simulink model "basic_charging_arm"  (R2022b)
settings: Solver=VariableStepAuto  StartTime=0.0  StopTime=100  RelTol=1e-3
values from neighbouring files (symbols this model uses):
  X = zeros(3,1)    [fk.m]
undefined symbols (not defined in the file or in its folder): Y, Z
libraries: fl_lib x64, fl_ps_legacy_lib x32, nesl_utility x25, sm_lib x24, simulink_extras x8, ee_lib x8, simulink x4, slpidlib x4, robotcorelib x1, robotmaniplib x1
(part 1 of 3)
settings Model: Creator=Mohit  LastModifiedBy=Mohit

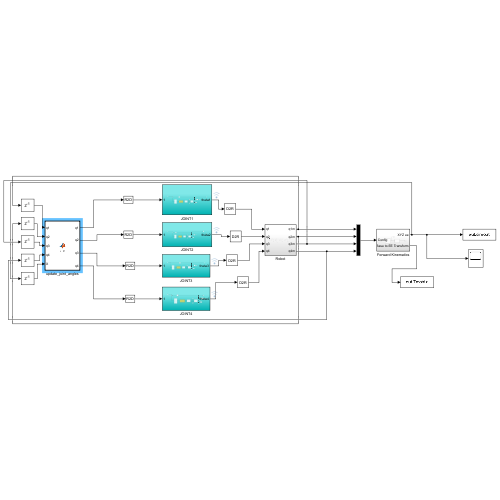
[thumbnail: Simulink's stored preview of the top-level diagram]
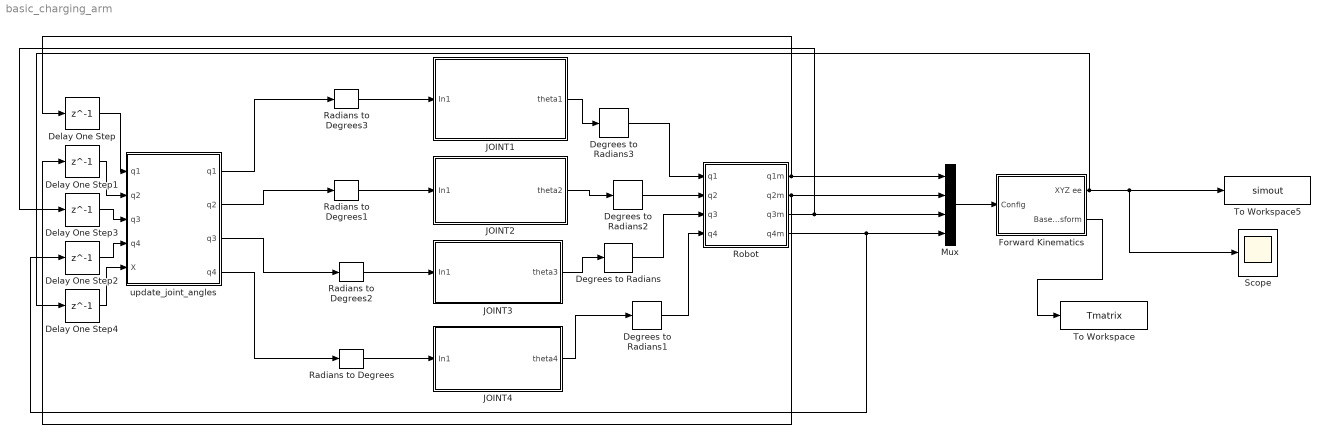
== system basic_charging_arm ==
  Degrees to Radians{,1..3} (4 alike) : simulink_extras/Transformations/Degrees to Radians
  Delay One Step{,1..4} (5 alike) : Delay  DelayLength=1
  Forward Kinematics : Subsystem
  JOINT1 : Subsystem
  JOINT2 : Subsystem
  JOINT3 : Subsystem
  JOINT4 : Subsystem
  Mux : Mux
  Radians to Degrees{,1..3} (4 alike) : simulink_extras/Transformations/Radians to Degrees
  Robot : Subsystem
  Scope : Scope
  To Workspace : ToWorkspace  VariableName=Tmatrix  SaveFormat=Timeseries  SampleTime=-1
  To Workspace5 : ToWorkspace  VariableName=simout  SaveFormat=Timeseries  SampleTime=-1
  update_joint_angles : MATLAB Function  TreatAsAtomicUnit=on
  wires:
  Mux/1 -> Forward Kinematics/1(Config)
  Forward Kinematics/2(Base to EE Transform) -> To Workspace/1
  Robot/1(q1m) -> Delay One Step/1, Mux/1
  Robot/2(q2m) -> Delay One Step1/1, Mux/2
  Robot/3(q3m) -> Delay One Step3/1, Mux/3
  Robot/4(q4m) -> Delay One Step2/1, Mux/4
  Radians to Degrees/1 -> JOINT4/1(In1)
  Radians to Degrees1/1 -> JOINT2/1(In1)
  Radians to Degrees3/1 -> JOINT1/1(In1)
  JOINT1/1(theta1) -> Degrees to Radians3/1
  Forward Kinematics/1(XYZ ee) -> Delay One Step4/1, To Workspace5/1, Scope/1
  JOINT3/1(theta3) -> Degrees to Radians/1
  JOINT4/1(theta4) -> Degrees to Radians1/1
  Radians to Degrees2/1 -> JOINT3/1(In1)
  JOINT2/1(theta2) -> Degrees to Radians2/1
  Degrees to Radians1/1 -> Robot/4(q4)
  Degrees to Radians3/1 -> Robot/1(q1)
  Degrees to Radians2/1 -> Robot/2(q2)
  Degrees to Radians/1 -> Robot/3(q3)
  update_joint_angles/1(q1) -> Radians to Degrees3/1
  update_joint_angles/2(q2) -> Radians to Degrees1/1
  update_joint_angles/3(q3) -> Radians to Degrees2/1
  update_joint_angles/4(q4) -> Radians to Degrees/1
  Delay One Step/1 -> update_joint_angles/1("q1 ")
  Delay One Step2/1 -> update_joint_angles/4("q4 ")
  Delay One Step3/1 -> update_joint_angles/3("q3 ")
  Delay One Step1/1 -> update_joint_angles/2("q2 ")
  Delay One Step4/1 -> update_joint_angles/5(X)

== system basic_charging_arm/Forward Kinematics ==
  Config : Inport
  Coordinate Transformation Conversion : robotcorelib/Coordinate Transformation Conversion  InputRepresentation=Homogeneous Transformation  InputEulerSequence=ZYX  ShowTrVecInputPort=on  OutputRepresentation=Translation Vector  OutputEulerSequence=ZYX  ShowTrVecOutputPort=on  SimulateUsing=Interpreted execution
  Get Transform : robotmaniplib/Get Transform  RigidBodyTree=Basic_arm_rbt  SourceBody=Body5  TargetBody=Base  SimulateUsing=Interpreted execution
  XYZ ee : Outport
  Base to EE Transform : Outport  Port=2
  wires:
  Config/1 -> Get Transform/1
  Coordinate Transformation Conversion/1 -> XYZ ee/1  "XYZ ee"
  Get Transform/1 -> Base to EE Transform/1, Coordinate Transformation Conversion/1

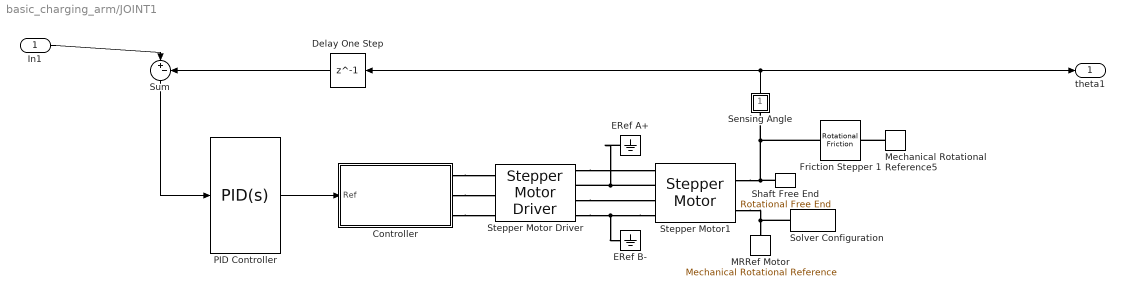
== system basic_charging_arm/JOINT1 ==
  In1 : Inport
  Controller : Subsystem  Variant=on  VariantControlMode=label  LabelModeActiveChoice=Speed
      settings: AttributesFormatString=%<BlockChoice>
  Delay One Step : Delay  DelayLength=1
  ERef A+ : fl_lib/Electrical/Electrical Elements/Electrical Reference
  ERef B- : fl_lib/Electrical/Electrical Elements/Electrical Reference
  Friction Stepper 1 : fl_lib/Mechanical/Rotational Elements/Rotational Friction  brkwy_trq=3.0e-2 N*m  brkwy_vel=0.03347 rad/s  Col_trq=3.0e-2 N*m  visc_coef=0 N*m/(rad/s)  w_specify=off  w_priority=High  w=0 rad/s  w_nominal_specify=off  w_nominal_unit=rad/s  w_nominal_value=1  t_specify=off  t_priority=High  t=0 N*m  t_nominal_specify=off  t_nominal_unit=N*m  t_nominal_value=1
  MRRef Motor : fl_lib/Mechanical/Rotational Elements/Mechanical Rotational Reference
  Mechanical Rotational Reference5 : fl_lib/Mechanical/Rotational Elements/Mechanical Rotational Reference
  PID Controller : slpidlib/PID Controller  Controller=PID  Form=Parallel  TimeDomain=Continuous-time  UseExternalTs=off  SampleTime=-1  IntegratorMethod=Forward Euler  FilterMethod=Forward Euler  ControllerParametersSource=internal  P=6  I=6  UseKiTs=off  D=0  N=100  UseFilter=on  TunerSelectOption=Transfer Function Based (PID Tuner App)  InitialConditionSource=internal  InitialConditionForIntegrator=0  InitialConditionForFilter=0  DifferentiatorICPrevScaledInput=0  ExternalReset=none  TrackingMode=off  Kt=1  LimitOutput=off  SatLimitsSource=internal  UpperSaturationLimit=inf  LowerSaturationLimit=-inf  LinearizeAsGain=on  AntiWindupMode=none  Kb=1  LimitIntegrator=off  UpperIntegratorSaturationLimit=inf  LowerIntegratorSaturationLimit=-inf  POutMin=[]  POutMax=[]  IOutMin=[]  IOutMax=[]  DOutMin=[]  DOutMax=[]  NOutMin=[]  NOutMax=[]  SumOutMin=[]  SumOutMax=[]  SaturationOutMin=[]  SaturationOutMax=[]  PParamMin=[]  PParamMax=[]  IParamMin=[]  IParamMax=[]  DParamMin=[]  DParamMax=[]  NParamMin=[]  NParamMax=[]  KbParamMin=[]  KbParamMax=[]  KtParamMin=[]  KtParamMax=[]  KbOutMin=[]  KbOutMax=[]  KtOutMin=[]  KtOutMax=[]  IntegratorOutMin=[]  IntegratorOutMax=[]  FilterOutMin=[]  FilterOutMax=[]  SumI1OutMin=[]  SumI1OutMax=[]  SumI2OutMin=[]  SumI2OutMax=[]  SumI3OutMin=[]  SumI3OutMax=[]  SumI4OutMin=[]  SumI4OutMax=[]  SumDOutMin=[]  SumDOutMax=[]  DifferentiatorOutMin=[]  DifferentiatorOutMax=[]  FilterDiffOutCoefMin=[]  FilterDiffOutCoefMax=[]  ReciprocalOutMin=[]  ReciprocalOutMax=[]  SumDenOutMin=[]  SumDenOutMax=[]  SumNumOutMin=[]  SumNumOutMax=[]  DivideOutMin=[]  DivideOutMax=[]  UdiffTsProdOutMin=[]  UdiffTsProdOutMax=[]  NTsProdOutMin=[]  NTsProdOutMax=[]  UintegralTsProdOutMin=[]  UintegralTsProdOutMax=[]  UngainTsProdOutMin=[]  UngainTsProdOutMax=[]  ClampingZeroOutDataTypeStr=Inherit: Inherit via back propagation  ClampingZeroOutMin=[]  ClampingZeroOutMax=[]  FilterDenConstantOutDataTypeStr=Inherit: Inherit via back propagation  FilterDenConstantOutMin=[]  FilterDenConstantOutMax=[]  PCopyOutDataTypeStr=Inherit: Inherit via back propagation  PCopyOutMin=[]  PCopyOutMax=[]  NCopyOutDataTypeStr=Inherit: Inherit via back propagation  NCopyOutMin=[]  NCopyOutMax=[]  IntegratorContinuousStateAttributes=''  IntegratorStateMustResolveToSignalObject=off  IntegratorRTWStateStorageClass=Auto  FilterContinuousStateAttributes=''  FilterStateMustResolveToSignalObject=off  FilterRTWStateStorageClass=Auto  ParallelPVariant=InternalParameters  IdealPVariant=Disabled  IVariant=InternalParameters  DVariant=InternalParameters  IntegratorVariant=Continuous  SatVariant=Disabled  AWVariant=Passthrough  PCopyVariant=Disabled  TRVariant=Disabled  FdbkBlocksVariant=Forward  IdealPFdbkVariant=Disabled  SatFdbkVariant=Disabled  DerivativeFilterVariant=ContFilter  NVariant=InternalParameters  NCopyVariant=Disabled  FilterICVariant=InternalICsFilter  IntegratorICVariant=InternalICs  ExternalResetVariant=Disabled  TRSumVariant=Passthrough  SumFdbkVariant=Disabled  SumVariant=Sum_PID  TsampFilterVariant=InternalTs  TsampNgainVariant=Passthrough  TsampIntegralVariant=Passthrough  ExternalSaturationOutDataTypeStr=Inherit: Same as second input
  Sensing Angle : Subsystem
      mask Display: disp('a')
  Shaft Free End : fl_lib/Mechanical/Rotational Elements/Rotational Free End  w_specify=off  w_priority=None  w=0 rad/s  w_nominal_specify=off  w_nominal_unit=rad/s  w_nominal_value=1
  Solver Configuration : nesl_utility/Solver Configuration  PhysicalDomain=network_engine_domain  SubClassName=solver  LeftPortType=input  RightPortType=generic  Tones=[]  Harmonics=[]  SimulateNoise=off  Profile=off  UseLocalSampling=off  EnableSwitchedLinearOptims=on  FrequencyDomain=off  UseCCode=off  RelTol=0.001  AbsTol=1e-06  MinStep=1e-09  ToWorkspace=off  RevertToSquareIcSolve=off  NumHomotopyIterations=100  PhasorMode=off  PhasorModeNumHarmonics=1  ConsistencySolver=NEWTON_FTOL  IndexReductionMethod=DerivativeReplacement  DoDC=off  ResidualTolerance=1e-9  ConsistencyTolSource=GLOBAL  ConsistencyAbsTol=0.001  ConsistencyRelTol=0.001  ConsistencyTolFactor=0.001  UseLocalSolver=off  LocalSolverChoice=NE_BACKWARD_EULER_ADVANCER  ResolveIndetEquations=on  FunctionEvalNumThread=1  LocalSolverSampleTime=.001  DoFixedCost=off  MaxNonlinIter=3  MaxModeIter=2  ComputeImpulses=off  ImpulseIterations=2  LinearAlgebra=auto  LinearAlgebraNumThread=0  EquationFormulation=NE_TIME_EF  DelaysMemoryBudget=1024  AutomaticFiltering=on  FilteringTimeConstant=0.001  PartitionStorageMethod=AS_NEEDED  PartitionMemoryBudget=1024  PartitionMethod=FAST
  Stepper Motor Driver : ee_lib/Electromechanical/Reluctance & Stepper/Stepper Motor Driver  step_or_av=ee.enum.electromech.simulationMode.stepping  step_rate_per_volt=10 Hz/V  Venable=2.5 V  Vreverse=2.5 V  supply_ports=ee.enum.supply_ports.hidesupply  Vm=5 V  Vsupply=10 V  half_stepping=ee.enum.electromech.steppingModeAveraged.fullStep  stepping_mode=ee.enum.electromech.steppingMode.microStep  numMicroSteps=4  Im=1.2 A
      settings: InternalSimscapePortConfiguration="{\"Bottom\":[],\"Left\":[{\"id\":\"ENA\",\"label\":\"ENA\",\"type\":\"foundation.electrical.electrical\"},{\"id\":\"REF\",\"label\":\"REF\",\"type\":\"foundation.electrical.electrical\"},{\"id\":\"REV\",\"label\":\"REV\",\"type\":\"foundation.electrical.electrical\"}],\"Right\":[{\"id\":\"pA\",\"label\":\"A+\",\"type\":\"foundation.electrical.electrical\"},{\"id\":\"nA\",\"label\":\"A-\",\"type\":\"foundation.electrical.electrical\"},{\"id\":\"pB\",\"label\":\"B+\",\"type\":\"foundation.electrical.electrical\"},{\"id\":\"nB\",\"label\":\"B-\",\"type\":\"foundation.electrical.electrical\"}],\"Top\":[]}"
  Stepper Motor1 : ee_lib/Electromechanical/Reluctance & Stepper/Stepper Motor  step_or_av=1  Ra=0.55 Ohm  La=0.0015 H  Km=0.19 N*m/A  Td=0 N*m  Rm=Inf Ohm  w_vec=[ 0 1000 3e+3 ] rpm  T_vec=[ 2 2 1 ] N*m  assert_if_slipping=0  J_total=1e-4 kg*m^2  max_step_rate=10 Hz  Step=1.8 deg  J=4.5e-05 kg*m^2  B=1e-02 N*m/(rad/s)  speed0=0 rpm  theta0=0 deg  alpha=[.00393, .00393] 1/K  Tmeas=25 degC  Tmeas2=125 degC  T_vec2=[1.7, 1.7, .85] N*m  half_stepping=ee.enum.electromech.steppingModeAveraged.fullStep  thermal_masses=[100, 100] J/K  initial_temperatures=[25, 25] degC  rotor_thermal_mass=50 J/K  rotor_initial_temperature=25 degC  Rm_percent_rotor=90
      settings: InternalSimscapePortConfiguration="{\"Bottom\":[],\"Left\":[{\"id\":\"pA\",\"label\":\"A+\",\"type\":\"foundation.electrical.electrical\"},{\"id\":\"nA\",\"label\":\"A-\",\"type\":\"foundation.electrical.electrical\"},{\"id\":\"pB\",\"label\":\"B+\",\"type\":\"foundation.electrical.electrical\"},{\"id\":\"nB\",\"label\":\"B-\",\"type\":\"foundation.electrical.electrical\"}],\"Right\":[{\"id\":\"R\",\"label\":\"R\",\"type\":\"foundation.mechanical.rotational.rotational\"},{\"id\":\"C\",\"label\":\"C\",\"type\":\"foundation.mechanical.rotational.rotational\"}],\"Top\":[]}"
  Sum : Sum  Inputs=|+-
  theta1 : Outport
  wires:
  In1/1 -> Sum/1
  Sum/1 -> PID Controller/1
  Sensing Angle/1(theta) -> theta1/1, Delay One Step/1
  PID Controller/1 -> Controller/1(Ref)
  Delay One Step/1 -> Sum/2
  connections:
  Controller/RConn2 -- Stepper Motor Driver/LConn2
  Stepper Motor Driver/RConn1 -- Stepper Motor1/LConn1
  Controller/RConn1 -- Stepper Motor Driver/LConn1
  Solver Configuration/RConn1 -- Stepper Motor1/RConn2 -- MRRef Motor/LConn1
  ERef A+/LConn1 -- Stepper Motor1/LConn2 -- Stepper Motor Driver/RConn2
  Stepper Motor Driver/RConn3 -- Stepper Motor1/LConn3
  Mechanical Rotational Reference5/LConn1 -- Friction Stepper 1/RConn1
  Controller/RConn3 -- Stepper Motor Driver/LConn3
  Stepper Motor1/LConn4 -- Stepper Motor Driver/RConn4 -- ERef B-/LConn1
  Sensing Angle/LConn1 -- Friction Stepper 1/LConn1 -- Shaft Free End/LConn1 -- Stepper Motor1/RConn1

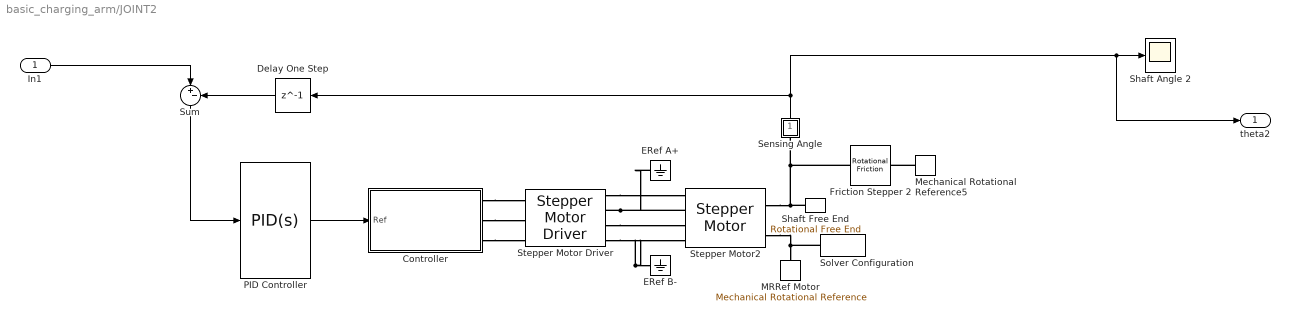
== system basic_charging_arm/JOINT2 ==
  In1 : Inport
  Controller : Subsystem  Variant=on  VariantControlMode=label  LabelModeActiveChoice=Speed
      settings: AttributesFormatString=%<BlockChoice>
  Delay One Step : Delay  DelayLength=1
  ERef A+ : fl_lib/Electrical/Electrical Elements/Electrical Reference
  ERef B- : fl_lib/Electrical/Electrical Elements/Electrical Reference
  Friction Stepper 2 : fl_lib/Mechanical/Rotational Elements/Rotational Friction  brkwy_trq=3.0e-2 N*m  brkwy_vel=0.03347 rad/s  Col_trq=3.0e-2 N*m  visc_coef=0 N*m/(rad/s)  w_specify=off  w_priority=High  w=0 rad/s  w_nominal_specify=off  w_nominal_unit=rad/s  w_nominal_value=1  t_specify=off  t_priority=High  t=0 N*m  t_nominal_specify=off  t_nominal_unit=N*m  t_nominal_value=1
  MRRef Motor : fl_lib/Mechanical/Rotational Elements/Mechanical Rotational Reference
  Mechanical Rotational Reference5 : fl_lib/Mechanical/Rotational Elements/Mechanical Rotational Reference
  PID Controller : slpidlib/PID Controller  Controller=PID  Form=Parallel  TimeDomain=Continuous-time  UseExternalTs=off  SampleTime=-1  IntegratorMethod=Forward Euler  FilterMethod=Forward Euler  ControllerParametersSource=internal  P=6  I=6  UseKiTs=off  D=0  N=100  UseFilter=on  TunerSelectOption=Transfer Function Based (PID Tuner App)  InitialConditionSource=internal  InitialConditionForIntegrator=0  InitialConditionForFilter=0  DifferentiatorICPrevScaledInput=0  ExternalReset=none  TrackingMode=off  Kt=1  LimitOutput=off  SatLimitsSource=internal  UpperSaturationLimit=inf  LowerSaturationLimit=-inf  LinearizeAsGain=on  AntiWindupMode=none  Kb=1  LimitIntegrator=off  UpperIntegratorSaturationLimit=inf  LowerIntegratorSaturationLimit=-inf  POutMin=[]  POutMax=[]  IOutMin=[]  IOutMax=[]  DOutMin=[]  DOutMax=[]  NOutMin=[]  NOutMax=[]  SumOutMin=[]  SumOutMax=[]  SaturationOutMin=[]  SaturationOutMax=[]  PParamMin=[]  PParamMax=[]  IParamMin=[]  IParamMax=[]  DParamMin=[]  DParamMax=[]  NParamMin=[]  NParamMax=[]  KbParamMin=[]  KbParamMax=[]  KtParamMin=[]  KtParamMax=[]  KbOutMin=[]  KbOutMax=[]  KtOutMin=[]  KtOutMax=[]  IntegratorOutMin=[]  IntegratorOutMax=[]  FilterOutMin=[]  FilterOutMax=[]  SumI1OutMin=[]  SumI1OutMax=[]  SumI2OutMin=[]  SumI2OutMax=[]  SumI3OutMin=[]  SumI3OutMax=[]  SumI4OutMin=[]  SumI4OutMax=[]  SumDOutMin=[]  SumDOutMax=[]  DifferentiatorOutMin=[]  DifferentiatorOutMax=[]  FilterDiffOutCoefMin=[]  FilterDiffOutCoefMax=[]  ReciprocalOutMin=[]  ReciprocalOutMax=[]  SumDenOutMin=[]  SumDenOutMax=[]  SumNumOutMin=[]  SumNumOutMax=[]  DivideOutMin=[]  DivideOutMax=[]  UdiffTsProdOutMin=[]  UdiffTsProdOutMax=[]  NTsProdOutMin=[]  NTsProdOutMax=[]  UintegralTsProdOutMin=[]  UintegralTsProdOutMax=[]  UngainTsProdOutMin=[]  UngainTsProdOutMax=[]  ClampingZeroOutDataTypeStr=Inherit: Inherit via back propagation  ClampingZeroOutMin=[]  ClampingZeroOutMax=[]  FilterDenConstantOutDataTypeStr=Inherit: Inherit via back propagation  FilterDenConstantOutMin=[]  FilterDenConstantOutMax=[]  PCopyOutDataTypeStr=Inherit: Inherit via back propagation  PCopyOutMin=[]  PCopyOutMax=[]  NCopyOutDataTypeStr=Inherit: Inherit via back propagation  NCopyOutMin=[]  NCopyOutMax=[]  IntegratorContinuousStateAttributes=''  IntegratorStateMustResolveToSignalObject=off  IntegratorRTWStateStorageClass=Auto  FilterContinuousStateAttributes=''  FilterStateMustResolveToSignalObject=off  FilterRTWStateStorageClass=Auto  ParallelPVariant=InternalParameters  IdealPVariant=Disabled  IVariant=InternalParameters  DVariant=InternalParameters  IntegratorVariant=Continuous  SatVariant=Disabled  AWVariant=Passthrough  PCopyVariant=Disabled  TRVariant=Disabled  FdbkBlocksVariant=Forward  IdealPFdbkVariant=Disabled  SatFdbkVariant=Disabled  DerivativeFilterVariant=ContFilter  NVariant=InternalParameters  NCopyVariant=Disabled  FilterICVariant=InternalICsFilter  IntegratorICVariant=InternalICs  ExternalResetVariant=Disabled  TRSumVariant=Passthrough  SumFdbkVariant=Disabled  SumVariant=Sum_PID  TsampFilterVariant=InternalTs  TsampNgainVariant=Passthrough  TsampIntegralVariant=Passthrough  ExternalSaturationOutDataTypeStr=Inherit: Same as second input
  Sensing Angle : Subsystem
      mask Display: disp('a')
  Shaft Angle 2 : Scope
  Shaft Free End : fl_lib/Mechanical/Rotational Elements/Rotational Free End  w_specify=off  w_priority=None  w=0 rad/s  w_nominal_specify=off  w_nominal_unit=rad/s  w_nominal_value=1
  Solver Configuration : nesl_utility/Solver Configuration  PhysicalDomain=network_engine_domain  SubClassName=solver  LeftPortType=input  RightPortType=generic  Tones=[]  Harmonics=[]  SimulateNoise=off  Profile=off  UseLocalSampling=off  EnableSwitchedLinearOptims=on  FrequencyDomain=off  UseCCode=off  RelTol=0.001  AbsTol=1e-06  MinStep=1e-09  ToWorkspace=off  RevertToSquareIcSolve=off  NumHomotopyIterations=100  PhasorMode=off  PhasorModeNumHarmonics=1  ConsistencySolver=NEWTON_FTOL  IndexReductionMethod=DerivativeReplacement  DoDC=off  ResidualTolerance=1e-9  ConsistencyTolSource=GLOBAL  ConsistencyAbsTol=0.001  ConsistencyRelTol=0.001  ConsistencyTolFactor=0.001  UseLocalSolver=off  LocalSolverChoice=NE_BACKWARD_EULER_ADVANCER  ResolveIndetEquations=on  FunctionEvalNumThread=1  LocalSolverSampleTime=.001  DoFixedCost=off  MaxNonlinIter=3  MaxModeIter=2  ComputeImpulses=off  ImpulseIterations=2  LinearAlgebra=auto  LinearAlgebraNumThread=0  EquationFormulation=NE_TIME_EF  DelaysMemoryBudget=1024  AutomaticFiltering=on  FilteringTimeConstant=0.001  PartitionStorageMethod=AS_NEEDED  PartitionMemoryBudget=1024  PartitionMethod=FAST
  Stepper Motor Driver : ee_lib/Electromechanical/Reluctance & Stepper/Stepper Motor Driver  step_or_av=ee.enum.electromech.simulationMode.stepping  step_rate_per_volt=10 Hz/V  Venable=2.5 V  Vreverse=2.5 V  supply_ports=ee.enum.supply_ports.hidesupply  Vm=5 V  Vsupply=10 V  half_stepping=ee.enum.electromech.steppingModeAveraged.fullStep  stepping_mode=ee.enum.electromech.steppingMode.microStep  numMicroSteps=4  Im=1.2 A
      settings: InternalSimscapePortConfiguration="{\"Bottom\":[],\"Left\":[{\"id\":\"ENA\",\"label\":\"ENA\",\"type\":\"foundation.electrical.electrical\"},{\"id\":\"REF\",\"label\":\"REF\",\"type\":\"foundation.electrical.electrical\"},{\"id\":\"REV\",\"label\":\"REV\",\"type\":\"foundation.electrical.electrical\"}],\"Right\":[{\"id\":\"pA\",\"label\":\"A+\",\"type\":\"foundation.electrical.electrical\"},{\"id\":\"nA\",\"label\":\"A-\",\"type\":\"foundation.electrical.electrical\"},{\"id\":\"pB\",\"label\":\"B+\",\"type\":\"foundation.electrical.electrical\"},{\"id\":\"nB\",\"label\":\"B-\",\"type\":\"foundation.electrical.electrical\"}],\"Top\":[]}"
  Stepper Motor2 : ee_lib/Electromechanical/Reluctance & Stepper/Stepper Motor  step_or_av=1  Ra=0.55 Ohm  La=0.0015 H  Km=0.19 N*m/A  Td=0 N*m  Rm=Inf Ohm  w_vec=[ 0 1000 3e+3 ] rpm  T_vec=[ 2 2 1 ] N*m  assert_if_slipping=0  J_total=1e-4 kg*m^2  max_step_rate=10 Hz  Step=1.8 deg  J=4.5e-05 kg*m^2  B=1e-02 N*m/(rad/s)  speed0=0 rpm  theta0=0 deg  alpha=[.00393, .00393] 1/K  Tmeas=25 degC  Tmeas2=125 degC  T_vec2=[1.7, 1.7, .85] N*m  half_stepping=ee.enum.electromech.steppingModeAveraged.fullStep  thermal_masses=[100, 100] J/K  initial_temperatures=[25, 25] degC  rotor_thermal_mass=50 J/K  rotor_initial_temperature=25 degC  Rm_percent_rotor=90
      settings: InternalSimscapePortConfiguration="{\"Bottom\":[],\"Left\":[{\"id\":\"pA\",\"label\":\"A+\",\"type\":\"foundation.electrical.electrical\"},{\"id\":\"nA\",\"label\":\"A-\",\"type\":\"foundation.electrical.electrical\"},{\"id\":\"pB\",\"label\":\"B+\",\"type\":\"foundation.electrical.electrical\"},{\"id\":\"nB\",\"label\":\"B-\",\"type\":\"foundation.electrical.electrical\"}],\"Right\":[{\"id\":\"R\",\"label\":\"R\",\"type\":\"foundation.mechanical.rotational.rotational\"},{\"id\":\"C\",\"label\":\"C\",\"type\":\"foundation.mechanical.rotational.rotational\"}],\"Top\":[]}"
  Sum : Sum  Inputs=|+-
  theta2 : Outport
  wires:
  PID Controller/1 -> Controller/1(Ref)
  Sensing Angle/1(theta) -> Delay One Step/1, theta2/1, Shaft Angle 2/1
  Sum/1 -> PID Controller/1
  In1/1 -> Sum/1
  Delay One Step/1 -> Sum/2
  connections:
  Stepper Motor2/RConn1 -- Shaft Free End/LConn1 -- Friction Stepper 2/LConn1 -- Sensing Angle/LConn1
  ERef B-/LConn1 -- Stepper Motor Driver/RConn4 -- Stepper Motor2/LConn4
  Controller/RConn3 -- Stepper Motor Driver/LConn3
  Mechanical Rotational Reference5/LConn1 -- Friction Stepper 2/RConn1
  Stepper Motor Driver/RConn3 -- Stepper Motor2/LConn3
  Stepper Motor Driver/RConn2 -- Stepper Motor2/LConn2 -- ERef A+/LConn1
  MRRef Motor/LConn1 -- Stepper Motor2/RConn2 -- Solver Configuration/RConn1
  Controller/RConn1 -- Stepper Motor Driver/LConn1
  Stepper Motor Driver/RConn1 -- Stepper Motor2/LConn1
  Controller/RConn2 -- Stepper Motor Driver/LConn2

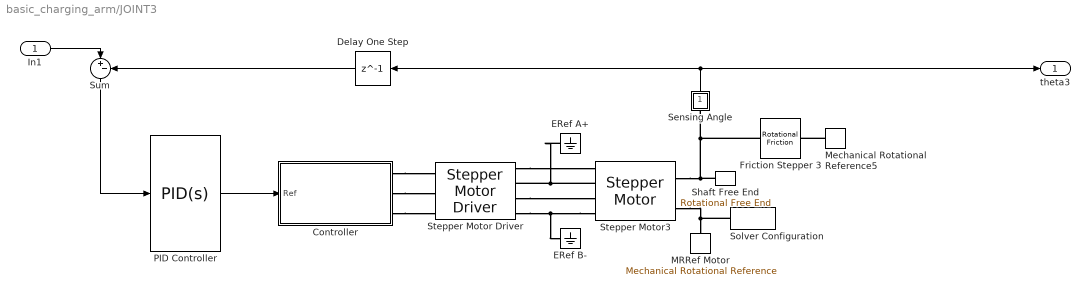
== system basic_charging_arm/JOINT3 ==
  In1 : Inport
  Controller : Subsystem  Variant=on  VariantControlMode=label  LabelModeActiveChoice=Speed
      settings: AttributesFormatString=%<BlockChoice>
  Delay One Step : Delay  DelayLength=1
  ERef A+ : fl_lib/Electrical/Electrical Elements/Electrical Reference
  ERef B- : fl_lib/Electrical/Electrical Elements/Electrical Reference
  Friction Stepper 3 : fl_lib/Mechanical/Rotational Elements/Rotational Friction  brkwy_trq=3.0e-2 N*m  brkwy_vel=0.03347 rad/s  Col_trq=3.0e-2 N*m  visc_coef=0 N*m/(rad/s)  w_specify=off  w_priority=High  w=0 rad/s  w_nominal_specify=off  w_nominal_unit=rad/s  w_nominal_value=1  t_specify=off  t_priority=High  t=0 N*m  t_nominal_specify=off  t_nominal_unit=N*m  t_nominal_value=1
  MRRef Motor : fl_lib/Mechanical/Rotational Elements/Mechanical Rotational Reference
  Mechanical Rotational Reference5 : fl_lib/Mechanical/Rotational Elements/Mechanical Rotational Reference
  PID Controller : slpidlib/PID Controller  Controller=PID  Form=Parallel  TimeDomain=Continuous-time  UseExternalTs=off  SampleTime=-1  IntegratorMethod=Forward Euler  FilterMethod=Forward Euler  ControllerParametersSource=internal  P=6  I=6  UseKiTs=off  D=0  N=100  UseFilter=on  TunerSelectOption=Transfer Function Based (PID Tuner App)  InitialConditionSource=internal  InitialConditionForIntegrator=0  InitialConditionForFilter=0  DifferentiatorICPrevScaledInput=0  ExternalReset=none  TrackingMode=off  Kt=1  LimitOutput=off  SatLimitsSource=internal  UpperSaturationLimit=inf  LowerSaturationLimit=-inf  LinearizeAsGain=on  AntiWindupMode=none  Kb=1  LimitIntegrator=off  UpperIntegratorSaturationLimit=inf  LowerIntegratorSaturationLimit=-inf  POutMin=[]  POutMax=[]  IOutMin=[]  IOutMax=[]  DOutMin=[]  DOutMax=[]  NOutMin=[]  NOutMax=[]  SumOutMin=[]  SumOutMax=[]  SaturationOutMin=[]  SaturationOutMax=[]  PParamMin=[]  PParamMax=[]  IParamMin=[]  IParamMax=[]  DParamMin=[]  DParamMax=[]  NParamMin=[]  NParamMax=[]  KbParamMin=[]  KbParamMax=[]  KtParamMin=[]  KtParamMax=[]  KbOutMin=[]  KbOutMax=[]  KtOutMin=[]  KtOutMax=[]  IntegratorOutMin=[]  IntegratorOutMax=[]  FilterOutMin=[]  FilterOutMax=[]  SumI1OutMin=[]  SumI1OutMax=[]  SumI2OutMin=[]  SumI2OutMax=[]  SumI3OutMin=[]  SumI3OutMax=[]  SumI4OutMin=[]  SumI4OutMax=[]  SumDOutMin=[]  SumDOutMax=[]  DifferentiatorOutMin=[]  DifferentiatorOutMax=[]  FilterDiffOutCoefMin=[]  FilterDiffOutCoefMax=[]  ReciprocalOutMin=[]  ReciprocalOutMax=[]  SumDenOutMin=[]  SumDenOutMax=[]  SumNumOutMin=[]  SumNumOutMax=[]  DivideOutMin=[]  DivideOutMax=[]  UdiffTsProdOutMin=[]  UdiffTsProdOutMax=[]  NTsProdOutMin=[]  NTsProdOutMax=[]  UintegralTsProdOutMin=[]  UintegralTsProdOutMax=[]  UngainTsProdOutMin=[]  UngainTsProdOutMax=[]  ClampingZeroOutDataTypeStr=Inherit: Inherit via back propagation  ClampingZeroOutMin=[]  ClampingZeroOutMax=[]  FilterDenConstantOutDataTypeStr=Inherit: Inherit via back propagation  FilterDenConstantOutMin=[]  FilterDenConstantOutMax=[]  PCopyOutDataTypeStr=Inherit: Inherit via back propagation  PCopyOutMin=[]  PCopyOutMax=[]  NCopyOutDataTypeStr=Inherit: Inherit via back propagation  NCopyOutMin=[]  NCopyOutMax=[]  IntegratorContinuousStateAttributes=''  IntegratorStateMustResolveToSignalObject=off  IntegratorRTWStateStorageClass=Auto  FilterContinuousStateAttributes=''  FilterStateMustResolveToSignalObject=off  FilterRTWStateStorageClass=Auto  ParallelPVariant=InternalParameters  IdealPVariant=Disabled  IVariant=InternalParameters  DVariant=InternalParameters  IntegratorVariant=Continuous  SatVariant=Disabled  AWVariant=Passthrough  PCopyVariant=Disabled  TRVariant=Disabled  FdbkBlocksVariant=Forward  IdealPFdbkVariant=Disabled  SatFdbkVariant=Disabled  DerivativeFilterVariant=ContFilter  NVariant=InternalParameters  NCopyVariant=Disabled  FilterICVariant=InternalICsFilter  IntegratorICVariant=InternalICs  ExternalResetVariant=Disabled  TRSumVariant=Passthrough  SumFdbkVariant=Disabled  SumVariant=Sum_PID  TsampFilterVariant=InternalTs  TsampNgainVariant=Passthrough  TsampIntegralVariant=Passthrough  ExternalSaturationOutDataTypeStr=Inherit: Same as second input
  Sensing Angle : Subsystem
      mask Display: disp('a')
  Shaft Free End : fl_lib/Mechanical/Rotational Elements/Rotational Free End  w_specify=off  w_priority=None  w=0 rad/s  w_nominal_specify=off  w_nominal_unit=rad/s  w_nominal_value=1
  Solver Configuration : nesl_utility/Solver Configuration  PhysicalDomain=network_engine_domain  SubClassName=solver  LeftPortType=input  RightPortType=generic  Tones=[]  Harmonics=[]  SimulateNoise=off  Profile=off  UseLocalSampling=off  EnableSwitchedLinearOptims=on  FrequencyDomain=off  UseCCode=off  RelTol=0.001  AbsTol=1e-06  MinStep=1e-09  ToWorkspace=off  RevertToSquareIcSolve=off  NumHomotopyIterations=100  PhasorMode=off  PhasorModeNumHarmonics=1  ConsistencySolver=NEWTON_FTOL  IndexReductionMethod=DerivativeReplacement  DoDC=off  ResidualTolerance=1e-9  ConsistencyTolSource=GLOBAL  ConsistencyAbsTol=0.001  ConsistencyRelTol=0.001  ConsistencyTolFactor=0.001  UseLocalSolver=off  LocalSolverChoice=NE_BACKWARD_EULER_ADVANCER  ResolveIndetEquations=on  FunctionEvalNumThread=1  LocalSolverSampleTime=.001  DoFixedCost=off  MaxNonlinIter=3  MaxModeIter=2  ComputeImpulses=off  ImpulseIterations=2  LinearAlgebra=auto  LinearAlgebraNumThread=0  EquationFormulation=NE_TIME_EF  DelaysMemoryBudget=1024  AutomaticFiltering=on  FilteringTimeConstant=0.001  PartitionStorageMethod=AS_NEEDED  PartitionMemoryBudget=1024  PartitionMethod=FAST
  Stepper Motor Driver : ee_lib/Electromechanical/Reluctance & Stepper/Stepper Motor Driver  step_or_av=ee.enum.electromech.simulationMode.stepping  step_rate_per_volt=10 Hz/V  Venable=2.5 V  Vreverse=2.5 V  supply_ports=ee.enum.supply_ports.hidesupply  Vm=5 V  Vsupply=10 V  half_stepping=ee.enum.electromech.steppingModeAveraged.fullStep  stepping_mode=ee.enum.electromech.steppingMode.microStep  numMicroSteps=4  Im=1.2 A
      settings: InternalSimscapePortConfiguration="{\"Bottom\":[],\"Left\":[{\"id\":\"ENA\",\"label\":\"ENA\",\"type\":\"foundation.electrical.electrical\"},{\"id\":\"REF\",\"label\":\"REF\",\"type\":\"foundation.electrical.electrical\"},{\"id\":\"REV\",\"label\":\"REV\",\"type\":\"foundation.electrical.electrical\"}],\"Right\":[{\"id\":\"pA\",\"label\":\"A+\",\"type\":\"foundation.electrical.electrical\"},{\"id\":\"nA\",\"label\":\"A-\",\"type\":\"foundation.electrical.electrical\"},{\"id\":\"pB\",\"label\":\"B+\",\"type\":\"foundation.electrical.electrical\"},{\"id\":\"nB\",\"label\":\"B-\",\"type\":\"foundation.electrical.electrical\"}],\"Top\":[]}"
  Stepper Motor3 : ee_lib/Electromechanical/Reluctance & Stepper/Stepper Motor  step_or_av=1  Ra=0.55 Ohm  La=0.0015 H  Km=0.19 N*m/A  Td=0 N*m  Rm=Inf Ohm  w_vec=[ 0 1000 3e+3 ] rpm  T_vec=[ 2 2 1 ] N*m  assert_if_slipping=0  J_total=1e-4 kg*m^2  max_step_rate=10 Hz  Step=1.8 deg  J=4.5e-05 kg*m^2  B=1e-02 N*m/(rad/s)  speed0=0 rpm  theta0=0 deg  alpha=[.00393, .00393] 1/K  Tmeas=25 degC  Tmeas2=125 degC  T_vec2=[1.7, 1.7, .85] N*m  half_stepping=ee.enum.electromech.steppingModeAveraged.fullStep  thermal_masses=[100, 100] J/K  initial_temperatures=[25, 25] degC  rotor_thermal_mass=50 J/K  rotor_initial_temperature=25 degC  Rm_percent_rotor=90
      settings: InternalSimscapePortConfiguration="{\"Bottom\":[],\"Left\":[{\"id\":\"pA\",\"label\":\"A+\",\"type\":\"foundation.electrical.electrical\"},{\"id\":\"nA\",\"label\":\"A-\",\"type\":\"foundation.electrical.electrical\"},{\"id\":\"pB\",\"label\":\"B+\",\"type\":\"foundation.electrical.electrical\"},{\"id\":\"nB\",\"label\":\"B-\",\"type\":\"foundation.electrical.electrical\"}],\"Right\":[{\"id\":\"R\",\"label\":\"R\",\"type\":\"foundation.mechanical.rotational.rotational\"},{\"id\":\"C\",\"label\":\"C\",\"type\":\"foundation.mechanical.rotational.rotational\"}],\"Top\":[]}"
  Sum : Sum  Inputs=|+-
  theta3 : Outport
  wires:
  In1/1 -> Sum/1
  Sum/1 -> PID Controller/1
  Sensing Angle/1(theta) -> theta3/1, Delay One Step/1
  PID Controller/1 -> Controller/1(Ref)
  Delay One Step/1 -> Sum/2
  connections:
  Controller/RConn2 -- Stepper Motor Driver/LConn2
  Stepper Motor Driver/RConn1 -- Stepper Motor3/LConn1
  Controller/RConn1 -- Stepper Motor Driver/LConn1
  Solver Configuration/RConn1 -- Stepper Motor3/RConn2 -- MRRef Motor/LConn1
  ERef A+/LConn1 -- Stepper Motor3/LConn2 -- Stepper Motor Driver/RConn2
  Stepper Motor Driver/RConn3 -- Stepper Motor3/LConn3
  Mechanical Rotational Reference5/LConn1 -- Friction Stepper 3/RConn1
  Controller/RConn3 -- Stepper Motor Driver/LConn3
  Stepper Motor3/LConn4 -- Stepper Motor Driver/RConn4 -- ERef B-/LConn1
  Sensing Angle/LConn1 -- Friction Stepper 3/LConn1 -- Shaft Free End/LConn1 -- Stepper Motor3/RConn1

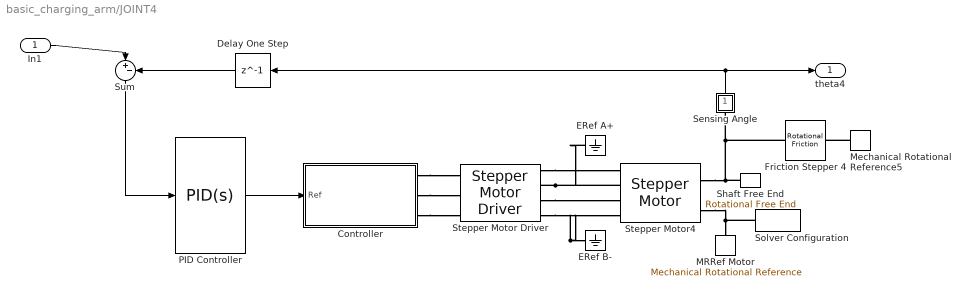
== system basic_charging_arm/JOINT4 ==
  In1 : Inport
  Controller : Subsystem  Variant=on  VariantControlMode=label  LabelModeActiveChoice=Speed
      settings: AttributesFormatString=%<BlockChoice>
  Delay One Step : Delay  DelayLength=1
  ERef A+ : fl_lib/Electrical/Electrical Elements/Electrical Reference
  ERef B- : fl_lib/Electrical/Electrical Elements/Electrical Reference
  Friction Stepper 4 : fl_lib/Mechanical/Rotational Elements/Rotational Friction  brkwy_trq=3.0e-2 N*m  brkwy_vel=0.03347 rad/s  Col_trq=3.0e-2 N*m  visc_coef=0 N*m/(rad/s)  w_specify=off  w_priority=High  w=0 rad/s  w_nominal_specify=off  w_nominal_unit=rad/s  w_nominal_value=1  t_specify=off  t_priority=High  t=0 N*m  t_nominal_specify=off  t_nominal_unit=N*m  t_nominal_value=1
  MRRef Motor : fl_lib/Mechanical/Rotational Elements/Mechanical Rotational Reference
  Mechanical Rotational Reference5 : fl_lib/Mechanical/Rotational Elements/Mechanical Rotational Reference
  PID Controller : slpidlib/PID Controller  Controller=PID  Form=Parallel  TimeDomain=Continuous-time  UseExternalTs=off  SampleTime=-1  IntegratorMethod=Forward Euler  FilterMethod=Forward Euler  ControllerParametersSource=internal  P=6  I=6  UseKiTs=off  D=0  N=100  UseFilter=on  TunerSelectOption=Transfer Function Based (PID Tuner App)  InitialConditionSource=internal  InitialConditionForIntegrator=0  InitialConditionForFilter=0  DifferentiatorICPrevScaledInput=0  ExternalReset=none  TrackingMode=off  Kt=1  LimitOutput=off  SatLimitsSource=internal  UpperSaturationLimit=inf  LowerSaturationLimit=-inf  LinearizeAsGain=on  AntiWindupMode=none  Kb=1  LimitIntegrator=off  UpperIntegratorSaturationLimit=inf  LowerIntegratorSaturationLimit=-inf  POutMin=[]  POutMax=[]  IOutMin=[]  IOutMax=[]  DOutMin=[]  DOutMax=[]  NOutMin=[]  NOutMax=[]  SumOutMin=[]  SumOutMax=[]  SaturationOutMin=[]  SaturationOutMax=[]  PParamMin=[]  PParamMax=[]  IParamMin=[]  IParamMax=[]  DParamMin=[]  DParamMax=[]  NParamMin=[]  NParamMax=[]  KbParamMin=[]  KbParamMax=[]  KtParamMin=[]  KtParamMax=[]  KbOutMin=[]  KbOutMax=[]  KtOutMin=[]  KtOutMax=[]  IntegratorOutMin=[]  IntegratorOutMax=[]  FilterOutMin=[]  FilterOutMax=[]  SumI1OutMin=[]  SumI1OutMax=[]  SumI2OutMin=[]  SumI2OutMax=[]  SumI3OutMin=[]  SumI3OutMax=[]  SumI4OutMin=[]  SumI4OutMax=[]  SumDOutMin=[]  SumDOutMax=[]  DifferentiatorOutMin=[]  DifferentiatorOutMax=[]  FilterDiffOutCoefMin=[]  FilterDiffOutCoefMax=[]  ReciprocalOutMin=[]  ReciprocalOutMax=[]  SumDenOutMin=[]  SumDenOutMax=[]  SumNumOutMin=[]  SumNumOutMax=[]  DivideOutMin=[]  DivideOutMax=[]  UdiffTsProdOutMin=[]  UdiffTsProdOutMax=[]  NTsProdOutMin=[]  NTsProdOutMax=[]  UintegralTsProdOutMin=[]  UintegralTsProdOutMax=[]  UngainTsProdOutMin=[]  UngainTsProdOutMax=[]  ClampingZeroOutDataTypeStr=Inherit: Inherit via back propagation  ClampingZeroOutMin=[]  ClampingZeroOutMax=[]  FilterDenConstantOutDataTypeStr=Inherit: Inherit via back propagation  FilterDenConstantOutMin=[]  FilterDenConstantOutMax=[]  PCopyOutDataTypeStr=Inherit: Inherit via back propagation  PCopyOutMin=[]  PCopyOutMax=[]  NCopyOutDataTypeStr=Inherit: Inherit via back propagation  NCopyOutMin=[]  NCopyOutMax=[]  IntegratorContinuousStateAttributes=''  IntegratorStateMustResolveToSignalObject=off  IntegratorRTWStateStorageClass=Auto  FilterContinuousStateAttributes=''  FilterStateMustResolveToSignalObject=off  FilterRTWStateStorageClass=Auto  ParallelPVariant=InternalParameters  IdealPVariant=Disabled  IVariant=InternalParameters  DVariant=InternalParameters  IntegratorVariant=Continuous  SatVariant=Disabled  AWVariant=Passthrough  PCopyVariant=Disabled  TRVariant=Disabled  FdbkBlocksVariant=Forward  IdealPFdbkVariant=Disabled  SatFdbkVariant=Disabled  DerivativeFilterVariant=ContFilter  NVariant=InternalParameters  NCopyVariant=Disabled  FilterICVariant=InternalICsFilter  IntegratorICVariant=InternalICs  ExternalResetVariant=Disabled  TRSumVariant=Passthrough  SumFdbkVariant=Disabled  SumVariant=Sum_PID  TsampFilterVariant=InternalTs  TsampNgainVariant=Passthrough  TsampIntegralVariant=Passthrough  ExternalSaturationOutDataTypeStr=Inherit: Same as second input
  Sensing Angle : Subsystem
      mask Display: disp('a')
  Shaft Free End : fl_lib/Mechanical/Rotational Elements/Rotational Free End  w_specify=off  w_priority=None  w=0 rad/s  w_nominal_specify=off  w_nominal_unit=rad/s  w_nominal_value=1
  Solver Configuration : nesl_utility/Solver Configuration  PhysicalDomain=network_engine_domain  SubClassName=solver  LeftPortType=input  RightPortType=generic  Tones=[]  Harmonics=[]  SimulateNoise=off  Profile=off  UseLocalSampling=off  EnableSwitchedLinearOptims=on  FrequencyDomain=off  UseCCode=off  RelTol=0.001  AbsTol=1e-06  MinStep=1e-09  ToWorkspace=off  RevertToSquareIcSolve=off  NumHomotopyIterations=100  PhasorMode=off  PhasorModeNumHarmonics=1  ConsistencySolver=NEWTON_FTOL  IndexReductionMethod=DerivativeReplacement  DoDC=off  ResidualTolerance=1e-9  ConsistencyTolSource=GLOBAL  ConsistencyAbsTol=0.001  ConsistencyRelTol=0.001  ConsistencyTolFactor=0.001  UseLocalSolver=off  LocalSolverChoice=NE_BACKWARD_EULER_ADVANCER  ResolveIndetEquations=on  FunctionEvalNumThread=1  LocalSolverSampleTime=.001  DoFixedCost=off  MaxNonlinIter=3  MaxModeIter=2  ComputeImpulses=off  ImpulseIterations=2  LinearAlgebra=auto  LinearAlgebraNumThread=0  EquationFormulation=NE_TIME_EF  DelaysMemoryBudget=1024  AutomaticFiltering=on  FilteringTimeConstant=0.001  PartitionStorageMethod=AS_NEEDED  PartitionMemoryBudget=1024  PartitionMethod=FAST
  Stepper Motor Driver : ee_lib/Electromechanical/Reluctance & Stepper/Stepper Motor Driver  step_or_av=ee.enum.electromech.simulationMode.stepping  step_rate_per_volt=10 Hz/V  Venable=2.5 V  Vreverse=2.5 V  supply_ports=ee.enum.supply_ports.hidesupply  Vm=5 V  Vsupply=10 V  half_stepping=ee.enum.electromech.steppingModeAveraged.fullStep  stepping_mode=ee.enum.electromech.steppingMode.microStep  numMicroSteps=4  Im=1.2 A
      settings: InternalSimscapePortConfiguration="{\"Bottom\":[],\"Left\":[{\"id\":\"ENA\",\"label\":\"ENA\",\"type\":\"foundation.electrical.electrical\"},{\"id\":\"REF\",\"label\":\"REF\",\"type\":\"foundation.electrical.electrical\"},{\"id\":\"REV\",\"label\":\"REV\",\"type\":\"foundation.electrical.electrical\"}],\"Right\":[{\"id\":\"pA\",\"label\":\"A+\",\"type\":\"foundation.electrical.electrical\"},{\"id\":\"nA\",\"label\":\"A-\",\"type\":\"foundation.electrical.electrical\"},{\"id\":\"pB\",\"label\":\"B+\",\"type\":\"foundation.electrical.electrical\"},{\"id\":\"nB\",\"label\":\"B-\",\"type\":\"foundation.electrical.electrical\"}],\"Top\":[]}"
  Stepper Motor4 : ee_lib/Electromechanical/Reluctance & Stepper/Stepper Motor  step_or_av=1  Ra=0.55 Ohm  La=0.0015 H  Km=0.19 N*m/A  Td=0 N*m  Rm=Inf Ohm  w_vec=[ 0 1000 3e+3 ] rpm  T_vec=[ 2 2 1 ] N*m  assert_if_slipping=0  J_total=1e-4 kg*m^2  max_step_rate=10 Hz  Step=1.8 deg  J=4.5e-05 kg*m^2  B=1e-02 N*m/(rad/s)  speed0=0 rpm  theta0=0 deg  alpha=[.00393, .00393] 1/K  Tmeas=25 degC  Tmeas2=125 degC  T_vec2=[1.7, 1.7, .85] N*m  half_stepping=ee.enum.electromech.steppingModeAveraged.fullStep  thermal_masses=[100, 100] J/K  initial_temperatures=[25, 25] degC  rotor_thermal_mass=50 J/K  rotor_initial_temperature=25 degC  Rm_percent_rotor=90
      settings: InternalSimscapePortConfiguration="{\"Bottom\":[],\"Left\":[{\"id\":\"pA\",\"label\":\"A+\",\"type\":\"foundation.electrical.electrical\"},{\"id\":\"nA\",\"label\":\"A-\",\"type\":\"foundation.electrical.electrical\"},{\"id\":\"pB\",\"label\":\"B+\",\"type\":\"foundation.electrical.electrical\"},{\"id\":\"nB\",\"label\":\"B-\",\"type\":\"foundation.electrical.electrical\"}],\"Right\":[{\"id\":\"R\",\"label\":\"R\",\"type\":\"foundation.mechanical.rotational.rotational\"},{\"id\":\"C\",\"label\":\"C\",\"type\":\"foundation.mechanical.rotational.rotational\"}],\"Top\":[]}"
  Sum : Sum  Inputs=|+-
  theta4 : Outport
  wires:
  PID Controller/1 -> Controller/1(Ref)
  Sensing Angle/1(theta) -> theta4/1, Delay One Step/1
  Sum/1 -> PID Controller/1
  In1/1 -> Sum/1
  Delay One Step/1 -> Sum/2
  connections:
  Stepper Motor4/RConn1 -- Shaft Free End/LConn1 -- Friction Stepper 4/LConn1 -- Sensing Angle/LConn1
  ERef B-/LConn1 -- Stepper Motor Driver/RConn4 -- Stepper Motor4/LConn4
  Controller/RConn3 -- Stepper Motor Driver/LConn3
  Mechanical Rotational Reference5/LConn1 -- Friction Stepper 4/RConn1
  Stepper Motor Driver/RConn3 -- Stepper Motor4/LConn3
  Stepper Motor Driver/RConn2 -- Stepper Motor4/LConn2 -- ERef A+/LConn1
  MRRef Motor/LConn1 -- Stepper Motor4/RConn2 -- Solver Configuration/RConn1
  Controller/RConn1 -- Stepper Motor Driver/LConn1
  Stepper Motor Driver/RConn1 -- Stepper Motor4/LConn1
  Controller/RConn2 -- Stepper Motor Driver/LConn2
